simulink model "zad2disc"  (R2014b)
settings: Solver=ode45  StartTime=0.0  StopTime=70  RelTol=1e-3
values from neighbouring files (symbols this model uses):
  a1 = -0.28    [set_params.m]
  a2 = -0.9    [set_params.m]
  a3 = 0.35    [set_params.m]
  a4 = 0.3    [set_params.m]
  K = 4.5    [set_params.m]
  T1 = 5    [set_params.m]
  T2 = 8    [set_params.m]
  Tp = 1    [zad10.m]    (also in zad11.m; zad3.m = Tp_vect(i); zad9.m)
settings Model: Creator=kuba  LastModifiedBy=kuba

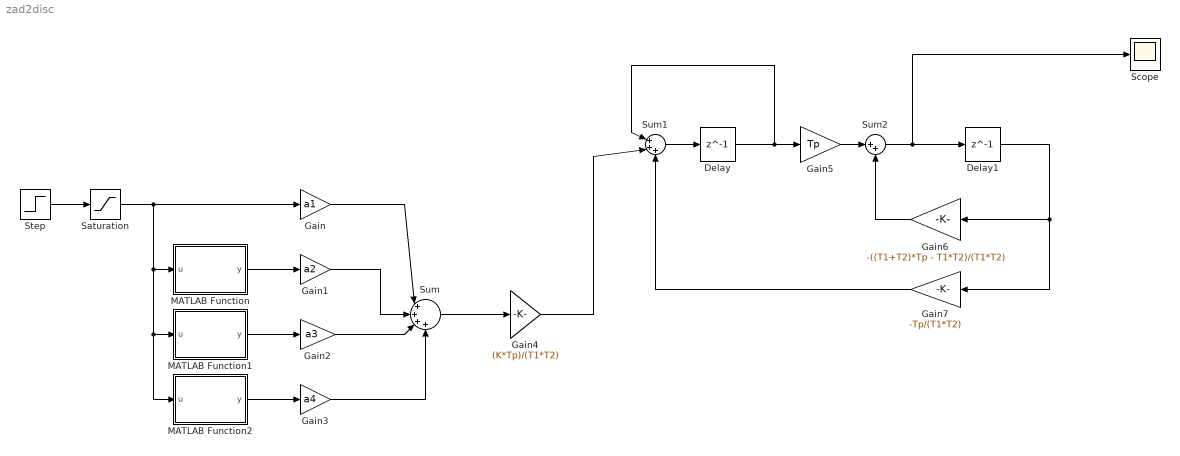
== system zad2disc ==
  Delay : Delay  DelayLength=1  InitialCondition=0  SampleTime=Tp
  Delay1 : Delay  DelayLength=1  InitialCondition=0  SampleTime=Tp
  Gain : Gain  Gain=a1  SampleTime=Tp
  Gain1 : Gain  Gain=a2  SampleTime=Tp
  Gain2 : Gain  Gain=a3  SampleTime=Tp
  Gain3 : Gain  Gain=a4  SampleTime=Tp
  Gain4 : Gain  Gain=(K*Tp)/(T1*T2)
  Gain5 : Gain  Gain=Tp
  Gain6 : Gain  Gain=-((T1+T2)*Tp - T1*T2)/(T1*T2)
  Gain7 : Gain  Gain=-Tp/(T1*T2)
  MATLAB Function : MATLAB Function  TreatAsAtomicUnit=on
  MATLAB Function1 : MATLAB Function  TreatAsAtomicUnit=on
  MATLAB Function2 : MATLAB Function  TreatAsAtomicUnit=on
  Saturation : Saturate  UpperLimit=1  LowerLimit=-1
  Scope : Scope
      settings: TimeRange=100  YMin=-1  YMax=1
  Step : Step  SampleTime=0
  Sum : Sum  Inputs=|++++
  Sum1 : Sum  Inputs=|+++
  Sum2 : Sum  Inputs=|++
  wires:
  Saturation/1 -> MATLAB Function2/1(u), MATLAB Function1/1(u), MATLAB Function/1(u), Gain/1
  MATLAB Function/1(y) -> Gain1/1
  MATLAB Function1/1(y) -> Gain2/1
  MATLAB Function2/1(y) -> Gain3/1
  Gain/1 -> Sum/1
  Gain1/1 -> Sum/2
  Gain2/1 -> Sum/3
  Gain3/1 -> Sum/4
  Sum/1 -> Gain4/1
  Step/1 -> Saturation/1
  Gain4/1 -> Sum1/2
  Sum1/1 -> Delay/1
  Delay/1 -> Gain5/1, Sum1/1
  Gain5/1 -> Sum2/1
  Sum2/1 -> Scope/1, Delay1/1
  Gain6/1 -> Sum2/2
  Gain7/1 -> Sum1/3
  Delay1/1 -> Gain7/1, Gain6/1

== matlab function zad2disc/MATLAB Function1 ==
  data: u input; y output
function y = cube(u)
y = u^3;

== matlab function zad2disc/MATLAB Function ==
  data: u input; y output
function y = square(u)
y = u^2;

== matlab function zad2disc/MATLAB Function2 ==
  data: u input; y output
function y = quad(u)
y = u^4;
